simulink model "test_view"  (R2015a)
settings: Solver=ode1  StartTime=0.0  StopTime=tmax  FixedStep=0.04  RelTol=1e-3
PostLoadFcn:
  | , if any(exist('dsrtsu_mdlpostloadfcn', 'file') == [2, 3, 6]), try dsrtsu_mdlpostloadfcn('Execute', bdroot); catch fprintf('Error in PostLoadFcn (dsrtsu_mdlpostloadfcn) for model "%s":\n %s\n', bdroot, lasterr); end, end,
libraries: vrlib x3
settings Model: DSRTSU_INTERNAL_RTI_VER=360  DSRTSU_INTERNAL_RTI_TYPE=rti1104  CovSFcnEnable=off  Creator=labor  LastModifiedBy=Schuettler
settings DataIOCC: SignalLoggingSaveFormat=ModelDataLogs
settings OptimizationCC: BlockReduction=off  OptimizeBlockIOStorage=off  BufferReuse=off  GlobalBufferReuse=off  ExpressionFolding=off  ExpressionDepthLimit=2147483647  LocalBlockOutputs=off  InitFltsAndDblsToZero=on  OptimizeModelRefInitCode=on  LifeSpan=1
settings DebuggingCC: UnderspecifiedInitializationDetection=Classic  MergeDetectMultiDrivingBlocksExec=none  SolverPrmCheckMsg=warning  FcnCallInpInsideContextMsg=UseLocalSettings  StateNameClashWarn=warning
settings HardwareCC: ProdIntDivRoundTo=Zero  ProdEndianess=BigEndian  ProdHWDeviceType=Generic->Custom  TargetIntDivRoundTo=Zero  TargetEndianess=BigEndian  TargetHWDeviceType=Generic->Custom
settings RTWCC: SystemTargetFile=ert.tlc  TemplateMakefile=ert_default_tmf  Description=Embedded Coder
settings CodeAppCC: IgnoreCustomStorageClasses=off
settings ERTTargetCC: ParMdlRefBuildCompliant=on  CompOptLevelCompliant=on  ConcurrentExecutionCompliant=on  ERTFirstTimeCompliant=on  SupportContinuousTime=off  SupportVariableSizeSignals=off  ModelStepFunctionPrototypeControlCompliant=on  CPPClassGenCompliant=on  InlinedParameterPlacement=Hierarchical  ERTCustomFileTemplate=example_file_process.tlc

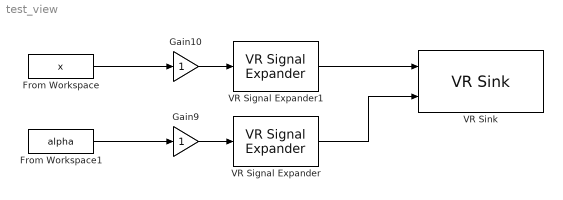
== system test_view ==
  From Workspace : FromWorkspace  VariableName=x  SampleTime=0
  From Workspace1 : FromWorkspace  VariableName=alpha  SampleTime=0
  Gain10 : Gain
  Gain9 : Gain
  VR Signal Expander : vrlib/VR Signal Expander  outwidth=4  outidx=[4]
  VR Signal Expander1 : vrlib/VR Signal Expander  outwidth=3  outidx=[1]
  VR Sink : vrlib/VR Sink  InstantiateOnLoad=on  SampleTime=-1  ViewEnable=on  RemoteChange=off  RemoteView=off  FieldsWritten=Wagen.translation.3.1.1.double#Pendelstabe.rotation.4.1.1.double  WorldFileName=invP.wrl  AutoView=off  VideoDimensions=[]  AllowVariableSize=off
  wires:
  Gain9/1 -> VR Signal Expander/1
  Gain10/1 -> VR Signal Expander1/1
  VR Signal Expander/1 -> VR Sink/2
  VR Signal Expander1/1 -> VR Sink/1
  From Workspace/1 -> Gain10/1
  From Workspace1/1 -> Gain9/1
